simulink model "kaiguangai1108"  (R2016b)
settings: Solver=ode4  StartTime=0.0  StopTime=inf  FixedStep=0.002  RelTol=1e-3  EnableMultiTasking=on
libraries: slrtlib x5
(part 5 of 6)

== stateflow chart kaiguangai1108/Subsystem1/shoudong/Chart3 ==
  state off
    en:
    skhx=0;
    kghx=0;
    gghx=0;
    yjhx=0;
    kgzhiling1=0;
    kgzhiling2=0;
    ggzhiling1=0;
    ggzhiling2=0;
    skyichang=0;
    kgyichang=0;
    sdyichang=0;
    jsyichang=0;
    ggyichang=0;
    yjyichang=0;
  state shoudong
    state songkai [parallel]
      settings: executionOrder=1
      state off
        entry:
        skhx=0;
      state on
        entry:
        skhx=1;
        skt=0;
        skyichang=0;
      state t
        entry:
        skt=skt+0.002;
      state t1
        entry:
        skyichang=1;
      state t2
        entry:
        skt=skt+0.002;
      (default) -> shoudong.songkai.off
      shoudong.songkai.t2 -> shoudong.songkai.off [order 2] : [skdw==1]
      (junction 19) -> shoudong.songkai.off [order 2] : [skdw==1&&skt<=2]
      shoudong.songkai.off -> shoudong.songkai.on : [songkai==1&&yjdw==1]
      shoudong.songkai.on -> (junction 19)
      (junction 19) -> shoudong.songkai.t1 [order 3] : [skt>2]
      shoudong.songkai.t -> (junction 19) : after(1,tick)
      (junction 19) -> shoudong.songkai.t [order 1] : [skdw==0&&skt<=2]
      shoudong.songkai.t1 -> shoudong.songkai.t2
      shoudong.songkai.t2 -> shoudong.songkai.t2 [order 1] : [skdw==0]
    state kaigai [parallel]
      settings: executionOrder=2
      state off
        entry:
        kghx=0;
        kgzhiling1=0;
        kgzhiling2=0；
      state on
        entry:
        kghx=1;
        kgzhiling1=1;
        kgzhiling2=1;
        kgyichang=0;
        kgt=0;
      state t
        entry:
        kgt=kgt+0.002;
      state t1
        entry:
        kgyichang=1;
      state t2
        entry:
        kgt=kgt+0.002;
      (default) -> shoudong.kaigai.off
      shoudong.kaigai.t2 -> shoudong.kaigai.off [order 2] : [kgdw1==1&&kgdw2==1]
      (junction 39) -> shoudong.kaigai.off [order 2] : [kgdw1==1&&kgdw2==1&&kgt<=12]
      shoudong.kaigai.off -> shoudong.kaigai.on : [kaigai==1&&skdw==1]
      shoudong.kaigai.on -> (junction 39)
      (junction 39) -> shoudong.kaigai.t1 [order 3] : [kgt>12]
      shoudong.kaigai.t -> (junction 39) : after(1,tick)
      (junction 39) -> shoudong.kaigai.t [order 1] : [(kgdw1==0||kgdw2==0)&&kgt<=12]
      shoudong.kaigai.t1 -> shoudong.kaigai.t2
      shoudong.kaigai.t2 -> shoudong.kaigai.t2 [order 1] : [kgdw1==0||kgdw2==0]
    state jiesuo_songkai [parallel]
      settings: executionOrder=4
      state off
        entry:
        skhx=0;
      state on
        entry:
        skhx=1;
        jsyichang=0;
        jst=0;
      state t
        entry:
        jst=jst+0.002;
      state t1
        entry:
        jsyichang=1;
      state t2
        entry:
        jst=jst+0.002;
      (default) -> shoudong.jiesuo_songkai.off
      shoudong.jiesuo_songkai.t2 -> shoudong.jiesuo_songkai.off [order 2] : [jsdw==1]
      (junction 60) -> shoudong.jiesuo_songkai.off [order 2] : [skdw==1&&jst<=2]
      shoudong.jiesuo_songkai.off -> shoudong.jiesuo_songkai.on : [jiesuo==1&&sddw==1]
      shoudong.jiesuo_songkai.on -> (junction 60)
      (junction 60) -> shoudong.jiesuo_songkai.t1 [order 3] : [jst>2]
      shoudong.jiesuo_songkai.t -> (junction 60) : after(1,tick)
      (junction 60) -> shoudong.jiesuo_songkai.t [order 1] : [jsdw==0&&jst<=2]
      shoudong.jiesuo_songkai.t1 -> shoudong.jiesuo_songkai.t2
      shoudong.jiesuo_songkai.t2 -> shoudong.jiesuo_songkai.t2 [order 1] : [jsdw==0]
    state suoding_yajin [parallel]
      settings: executionOrder=3
      state off
        entry:
        yjhx=0;
      state on
        entry:
        yjhx=1;
        sdyichang=0;
        sdt=0;
      state t1
        entry:
        sdyichang=1;
      state t2
        entry:
        sdt=sdt+0.002;
      state t
        entry:
        sdt=sdt+0.002;
      (default) -> shoudong.suoding_yajin.off
      shoudong.suoding_yajin.t2 -> shoudong.suoding_yajin.off [order 2] : [sddw==1]
      (junction 48) -> shoudong.suoding_yajin.off [order 2] : [sddw==1&&sdt<=2]
      shoudong.suoding_yajin.off -> shoudong.suoding_yajin.on : [suoding==1&&jsdw==1]
      shoudong.suoding_yajin.on -> (junction 48)
      (junction 48) -> shoudong.suoding_yajin.t1 [order 3] : [sdt>2]
      shoudong.suoding_yajin.t -> (junction 48) : after(1,tick)
      (junction 48) -> shoudong.suoding_yajin.t [order 1] : [sddw==0&&sdt<=2]
      shoudong.suoding_yajin.t1 -> shoudong.suoding_yajin.t2
      shoudong.suoding_yajin.t2 -> shoudong.suoding_yajin.t2 [order 1] : [sddw==0]
    state yajin [parallel]
      settings: executionOrder=6
      state off
        entry:
        yjhx=0;
      state on
        entry:
        yjhx=1;
        yjyichang=0;
        yjt=0;
      state t3
        entry:
        yjyichang=1;
      state t2
        entry:
        yjt=yjt+0.002;
      state t
        entry:
        yjt=yjt+0.002;
      (default) -> shoudong.yajin.off
      shoudong.yajin.t2 -> shoudong.yajin.off [order 2] : [yjdw==1]
      (junction 94) -> shoudong.yajin.off [order 2] : [yjdw==1&&sddw==1&&yjt<=2]
      shoudong.yajin.off -> shoudong.yajin.on : [yajin==1&&skdw==1]
      shoudong.yajin.on -> (junction 94)
      (junction 94) -> t3 [order 3] : [yjt>2]
      shoudong.yajin.t -> (junction 94) : after(1,tick)
      (junction 94) -> shoudong.yajin.t [order 1] : [yjdw==0&&yjt<=2]
      t3 -> shoudong.yajin.t2
      shoudong.yajin.t2 -> shoudong.yajin.t2 [order 1] : [yjdw==0]
    state guangai [parallel]
      settings: executionOrder=5
      state off
        entry:
        gghx=0;
        ggzhiling1=0;
        ggzhiling2=0
      state on
        entry:
        gghx=1;
        ggzhiling1=1;
        ggzhiling2=1;
        ggyichang=0;
        ggt=0;
      state t1
        entry:
        ggyichang=1;
      state t2
        entry:
        ggt=ggt+0.002;
      state t
        entry:
        ggt=ggt+0.002;
      (default) -> shoudong.guangai.off
      shoudong.guangai.t2 -> shoudong.guangai.off [order 2] : [ggdw1==1&&ggdw2==1]
      (junction 81) -> shoudong.guangai.off [order 2] : [ggdw1==1&&ggdw2==1&&ggt<=12]
      shoudong.guangai.off -> shoudong.guangai.on : [guangai==1&&kgdw1==1&&kgdw2==1]
      shoudong.guangai.on -> (junction 81)
      (junction 81) -> shoudong.guangai.t1 [order 3] : [ggt>12]
      shoudong.guangai.t -> (junction 81) : after(1,tick)
      (junction 81) -> shoudong.guangai.t [order 1] : [(ggdw1==0||ggdw2==0)&&ggt<=12]
      shoudong.guangai.t1 -> shoudong.guangai.t2
      shoudong.guangai.t2 -> shoudong.guangai.t2 [order 1] : [ggdw1==0||ggdw2==0]
  state off1
    en:
    skhx=0;
    kghx=0;
    gghx=0;
    yjhx=0;
    skt=0;
    kgt=0;
    sdt=0;
    jst=0;
    ggt=0;
    yjt=0;
    skyichang=0;
    kgyichang=0;
    sdyichang=0;
    jsyichang=0;
    ggyichang=0;
    yjyichang=0;
    kgzhiling1=0;
    kgzhiling2=0;
    ggzhiling1=0;
    ggzhiling2=0;
  (default) -> off
  off -> shoudong : [start==1&&jieshu==0]
  shoudong -> off1 : [jieshu==1]
  data: start input; kgdw1 input; kgdw2 input; ggdw1 input; ggdw2 input; sddw input; jsdw input; yjdw input; skdw input; songkai input; kaigai input; suoding input; jiesuo input; skhx output; kghx output; yjhx output; gghx output; kgzhiling1 output; kgzhiling2 output; ggzhiling1 output; ggzhiling2 output; skt output; kgt output; sdt output; jst output; ggt output; guangai input; yajin input; yjt output; skyichang output; kgyichang output; sdyichang output; jsyichang output; jieshu input; ggyichang output; yjyichang output

== stateflow chart kaiguangai1108/Subsystem1/shoudong/Chart4 ==
  state off
    en:
    skhx=0;
    kghx=0;
    gghx=0;
    yjhx=0;
    kgzhiling1=0;
    kgzhiling2=0;
    ggzhiling1=0;
    ggzhiling2=0;
    skyichang=0;
    kgyichang=0;
    sdyichang=0;
    jsyichang=0;
    ggyichang=0;
    yjyichang=0;
  state shoudong
    state songkai [parallel]
      settings: executionOrder=1
      state off
        entry:
        skhx=0;
      state on
        entry:
        skhx=1;
        skt=0;
        skyichang=0;
      state t
        entry:
        skt=skt+0.002;
      state t1
        entry:
        skyichang=1;
      state t2
        entry:
        skt=skt+0.002;
      (default) -> shoudong.songkai.off
      shoudong.songkai.t2 -> shoudong.songkai.off [order 2] : [skdw==1]
      (junction 19) -> shoudong.songkai.off [order 2] : [skdw==1&&skt<=2]
      shoudong.songkai.off -> shoudong.songkai.on : [songkai==1&&yjdw==1]
      shoudong.songkai.on -> (junction 19)
      (junction 19) -> shoudong.songkai.t1 [order 3] : [skt>2]
      shoudong.songkai.t -> (junction 19) : after(1,tick)
      (junction 19) -> shoudong.songkai.t [order 1] : [skdw==0&&skt<=2]
      shoudong.songkai.t1 -> shoudong.songkai.t2
      shoudong.songkai.t2 -> shoudong.songkai.t2 [order 1] : [skdw==0]
    state kaigai [parallel]
      settings: executionOrder=2
      state off
        entry:
        kghx=0;
        kgzhiling1=0;
        kgzhiling2=0；
      state on
        entry:
        kghx=1;
        kgzhiling1=1;
        kgzhiling2=1;
        kgyichang=0;
        kgt=0;
      state t
        entry:
        kgt=kgt+0.002;
      state t1
        entry:
        kgyichang=1;
      state t2
        entry:
        kgt=kgt+0.002;
      (default) -> shoudong.kaigai.off
      shoudong.kaigai.t2 -> shoudong.kaigai.off [order 2] : [kgdw1==1&&kgdw2==1]
      (junction 39) -> shoudong.kaigai.off [order 2] : [kgdw1==1&&kgdw2==1&&kgt<=12]
      shoudong.kaigai.off -> shoudong.kaigai.on : [kaigai==1&&skdw==1]
      shoudong.kaigai.on -> (junction 39)
      (junction 39) -> shoudong.kaigai.t1 [order 3] : [kgt>12]
      shoudong.kaigai.t -> (junction 39) : after(1,tick)
      (junction 39) -> shoudong.kaigai.t [order 1] : [(kgdw1==0||kgdw2==0)&&kgt<=12]
      shoudong.kaigai.t1 -> shoudong.kaigai.t2
      shoudong.kaigai.t2 -> shoudong.kaigai.t2 [order 1] : [kgdw1==0||kgdw2==0]
    state jiesuo_songkai [parallel]
      settings: executionOrder=4
      state off
        entry:
        skhx=0;
      state on
        entry:
        skhx=1;
        jsyichang=0;
        jst=0;
      state t
        entry:
        jst=jst+0.002;
      state t1
        entry:
        jsyichang=1;
      state t2
        entry:
        jst=jst+0.002;
      (default) -> shoudong.jiesuo_songkai.off
      shoudong.jiesuo_songkai.t2 -> shoudong.jiesuo_songkai.off [order 2] : [jsdw==1]
      (junction 60) -> shoudong.jiesuo_songkai.off [order 2] : [skdw==1&&jst<=2]
      shoudong.jiesuo_songkai.off -> shoudong.jiesuo_songkai.on : [jiesuo==1&&sddw==1]
      shoudong.jiesuo_songkai.on -> (junction 60)
      (junction 60) -> shoudong.jiesuo_songkai.t1 [order 3] : [jst>2]
      shoudong.jiesuo_songkai.t -> (junction 60) : after(1,tick)
      (junction 60) -> shoudong.jiesuo_songkai.t [order 1] : [jsdw==0&&jst<=2]
      shoudong.jiesuo_songkai.t1 -> shoudong.jiesuo_songkai.t2
      shoudong.jiesuo_songkai.t2 -> shoudong.jiesuo_songkai.t2 [order 1] : [jsdw==0]
    state suoding_yajin [parallel]
      settings: executionOrder=3
      state off
        entry:
        yjhx=0;
      state on
        entry:
        yjhx=1;
        sdyichang=0;
        sdt=0;
      state t1
        entry:
        sdyichang=1;
      state t2
        entry:
        sdt=sdt+0.002;
      state t
        entry:
        sdt=sdt+0.002;
      (default) -> shoudong.suoding_yajin.off
      shoudong.suoding_yajin.t2 -> shoudong.suoding_yajin.off [order 2] : [sddw==1]
      (junction 48) -> shoudong.suoding_yajin.off [order 2] : [sddw==1&&sdt<=2]
      shoudong.suoding_yajin.off -> shoudong.suoding_yajin.on : [suoding==1&&jsdw==1]
      shoudong.suoding_yajin.on -> (junction 48)
      (junction 48) -> shoudong.suoding_yajin.t1 [order 3] : [sdt>2]
      shoudong.suoding_yajin.t -> (junction 48) : after(1,tick)
      (junction 48) -> shoudong.suoding_yajin.t [order 1] : [sddw==0&&sdt<=2]
      shoudong.suoding_yajin.t1 -> shoudong.suoding_yajin.t2
      shoudong.suoding_yajin.t2 -> shoudong.suoding_yajin.t2 [order 1] : [sddw==0]
    state yajin [parallel]
      settings: executionOrder=6
      state off
        entry:
        yjhx=0;
      state on
        entry:
        yjhx=1;
        yjyichang=0;
        yjt=0;
      state t3
        entry:
        yjyichang=1;
      state t2
        entry:
        yjt=yjt+0.002;
      state t
        entry:
        yjt=yjt+0.002;
      (default) -> shoudong.yajin.off
      shoudong.yajin.t2 -> shoudong.yajin.off [order 2] : [yjdw==1]
      (junction 94) -> shoudong.yajin.off [order 2] : [yjdw==1&&sddw==1&&yjt<=2]
      shoudong.yajin.off -> shoudong.yajin.on : [yajin==1&&skdw==1]
      shoudong.yajin.on -> (junction 94)
      (junction 94) -> t3 [order 3] : [yjt>2]
      shoudong.yajin.t -> (junction 94) : after(1,tick)
      (junction 94) -> shoudong.yajin.t [order 1] : [yjdw==0&&yjt<=2]
      t3 -> shoudong.yajin.t2
      shoudong.yajin.t2 -> shoudong.yajin.t2 [order 1] : [yjdw==0]
    state guangai [parallel]
      settings: executionOrder=5
      state off
        entry:
        gghx=0;
        ggzhiling1=0;
        ggzhiling2=0
      state on
        entry:
        gghx=1;
        ggzhiling1=1;
        ggzhiling2=1;
        ggyichang=0;
        ggt=0;
      state t1
        entry:
        ggyichang=1;
      state t2
        entry:
        ggt=ggt+0.002;
      state t
        entry:
        ggt=ggt+0.002;
      (default) -> shoudong.guangai.off
      shoudong.guangai.t2 -> shoudong.guangai.off [order 2] : [ggdw1==1&&ggdw2==1]
      (junction 81) -> shoudong.guangai.off [order 2] : [ggdw1==1&&ggdw2==1&&ggt<=12]
      shoudong.guangai.off -> shoudong.guangai.on : [guangai==1&&kgdw1==1&&kgdw2==1]
      shoudong.guangai.on -> (junction 81)
      (junction 81) -> shoudong.guangai.t1 [order 3] : [ggt>12]
      shoudong.guangai.t -> (junction 81) : after(1,tick)
      (junction 81) -> shoudong.guangai.t [order 1] : [(ggdw1==0||ggdw2==0)&&ggt<=12]
      shoudong.guangai.t1 -> shoudong.guangai.t2
      shoudong.guangai.t2 -> shoudong.guangai.t2 [order 1] : [ggdw1==0||ggdw2==0]
  state off1
    en:
    skhx=0;
    kghx=0;
    gghx=0;
    yjhx=0;
    skt=0;
    kgt=0;
    sdt=0;
    jst=0;
    ggt=0;
    yjt=0;
    skyichang=0;
    kgyichang=0;
    sdyichang=0;
    jsyichang=0;
    ggyichang=0;
    yjyichang=0;
    kgzhiling1=0;
    kgzhiling2=0;
    ggzhiling1=0;
    ggzhiling2=0;
  (default) -> off
  off -> shoudong : [start==1&&jieshu==0]
  shoudong -> off1 : [jieshu==1]
  data: start input; kgdw1 input; kgdw2 input; ggdw1 input; ggdw2 input; sddw input; jsdw input; yjdw input; skdw input; songkai input; kaigai input; suoding input; jiesuo input; skhx output; kghx output; yjhx output; gghx output; kgzhiling1 output; kgzhiling2 output; ggzhiling1 output; ggzhiling2 output; skt output; kgt output; sdt output; jst output; ggt output; guangai input; yajin input; yjt output; skyichang output; kgyichang output; sdyichang output; jsyichang output; jieshu input; ggyichang output; yjyichang output

== stateflow chart kaiguangai1108/Subsystem1/shoudong/Chart5 ==
  state off
    en:
    skhx=0;
    kghx=0;
    gghx=0;
    yjhx=0;
    kgzhiling1=0;
    kgzhiling2=0;
    ggzhiling1=0;
    ggzhiling2=0;
    skyichang=0;
    kgyichang=0;
    sdyichang=0;
    jsyichang=0;
    ggyichang=0;
    yjyichang=0;
  state shoudong
    state songkai [parallel]
      settings: executionOrder=1
      state off
        entry:
        skhx=0;
      state on
        entry:
        skhx=1;
        skt=0;
        skyichang=0;
      state t
        entry:
        skt=skt+0.002;
      state t1
        entry:
        skyichang=1;
      state t2
        entry:
        skt=skt+0.002;
      (default) -> shoudong.songkai.off
      shoudong.songkai.t2 -> shoudong.songkai.off [order 2] : [skdw==1]
      (junction 19) -> shoudong.songkai.off [order 2] : [skdw==1&&skt<=2]
      shoudong.songkai.off -> shoudong.songkai.on : [songkai==1&&yjdw==1]
      shoudong.songkai.on -> (junction 19)
      (junction 19) -> shoudong.songkai.t1 [order 3] : [skt>2]
      shoudong.songkai.t -> (junction 19) : after(1,tick)
      (junction 19) -> shoudong.songkai.t [order 1] : [skdw==0&&skt<=2]
      shoudong.songkai.t1 -> shoudong.songkai.t2
      shoudong.songkai.t2 -> shoudong.songkai.t2 [order 1] : [skdw==0]
    state kaigai [parallel]
      settings: executionOrder=2
      state off
        entry:
        kghx=0;
        kgzhiling1=0;
        kgzhiling2=0；
      state on
        entry:
        kghx=1;
        kgzhiling1=1;
        kgzhiling2=1;
        kgyichang=0;
        kgt=0;
      state t
        entry:
        kgt=kgt+0.002;
      state t1
        entry:
        kgyichang=1;
      state t2
        entry:
        kgt=kgt+0.002;
      (default) -> shoudong.kaigai.off
      shoudong.kaigai.t2 -> shoudong.kaigai.off [order 2] : [kgdw1==1&&kgdw2==1]
      (junction 39) -> shoudong.kaigai.off [order 2] : [kgdw1==1&&kgdw2==1&&kgt<=12]
      shoudong.kaigai.off -> shoudong.kaigai.on : [kaigai==1&&skdw==1]
      shoudong.kaigai.on -> (junction 39)
      (junction 39) -> shoudong.kaigai.t1 [order 3] : [kgt>12]
      shoudong.kaigai.t -> (junction 39) : after(1,tick)
      (junction 39) -> shoudong.kaigai.t [order 1] : [(kgdw1==0||kgdw2==0)&&kgt<=12]
      shoudong.kaigai.t1 -> shoudong.kaigai.t2
      shoudong.kaigai.t2 -> shoudong.kaigai.t2 [order 1] : [kgdw1==0||kgdw2==0]
    state jiesuo_songkai [parallel]
      settings: executionOrder=4
      state off
        entry:
        skhx=0;
      state on
        entry:
        skhx=1;
        jsyichang=0;
        jst=0;
      state t
        entry:
        jst=jst+0.002;
      state t1
        entry:
        jsyichang=1;
      state t2
        entry:
        jst=jst+0.002;
      (default) -> shoudong.jiesuo_songkai.off
      shoudong.jiesuo_songkai.t2 -> shoudong.jiesuo_songkai.off [order 2] : [jsdw==1]
      (junction 60) -> shoudong.jiesuo_songkai.off [order 2] : [skdw==1&&jst<=2]
      shoudong.jiesuo_songkai.off -> shoudong.jiesuo_songkai.on : [jiesuo==1&&sddw==1]
      shoudong.jiesuo_songkai.on -> (junction 60)
      (junction 60) -> shoudong.jiesuo_songkai.t1 [order 3] : [jst>2]
      shoudong.jiesuo_songkai.t -> (junction 60) : after(1,tick)
      (junction 60) -> shoudong.jiesuo_songkai.t [order 1] : [jsdw==0&&jst<=2]
      shoudong.jiesuo_songkai.t1 -> shoudong.jiesuo_songkai.t2
      shoudong.jiesuo_songkai.t2 -> shoudong.jiesuo_songkai.t2 [order 1] : [jsdw==0]
    state suoding_yajin [parallel]
      settings: executionOrder=3
      state off
        entry:
        yjhx=0;
      state on
        entry:
        yjhx=1;
        sdyichang=0;
        sdt=0;
      state t1
        entry:
        sdyichang=1;
      state t2
        entry:
        sdt=sdt+0.002;
      state t
        entry:
        sdt=sdt+0.002;
      (default) -> shoudong.suoding_yajin.off
      shoudong.suoding_yajin.t2 -> shoudong.suoding_yajin.off [order 2] : [sddw==1]
      (junction 48) -> shoudong.suoding_yajin.off [order 2] : [sddw==1&&sdt<=2]
      shoudong.suoding_yajin.off -> shoudong.suoding_yajin.on : [suoding==1&&jsdw==1]
      shoudong.suoding_yajin.on -> (junction 48)
      (junction 48) -> shoudong.suoding_yajin.t1 [order 3] : [sdt>2]
      shoudong.suoding_yajin.t -> (junction 48) : after(1,tick)
      (junction 48) -> shoudong.suoding_yajin.t [order 1] : [sddw==0&&sdt<=2]
      shoudong.suoding_yajin.t1 -> shoudong.suoding_yajin.t2
      shoudong.suoding_yajin.t2 -> shoudong.suoding_yajin.t2 [order 1] : [sddw==0]
    state yajin [parallel]
      settings: executionOrder=6
      state off
        entry:
        yjhx=0;
      state on
        entry:
        yjhx=1;
        yjyichang=0;
        yjt=0;
      state t3
        entry:
        yjyichang=1;
      state t2
        entry:
        yjt=yjt+0.002;
      state t
        entry:
        yjt=yjt+0.002;
      (default) -> shoudong.yajin.off
      shoudong.yajin.t2 -> shoudong.yajin.off [order 2] : [yjdw==1]
      (junction 94) -> shoudong.yajin.off [order 2] : [yjdw==1&&sddw==1&&yjt<=2]
      shoudong.yajin.off -> shoudong.yajin.on : [yajin==1&&skdw==1]
      shoudong.yajin.on -> (junction 94)
      (junction 94) -> t3 [order 3] : [yjt>2]
      shoudong.yajin.t -> (junction 94) : after(1,tick)
      (junction 94) -> shoudong.yajin.t [order 1] : [yjdw==0&&yjt<=2]
      t3 -> shoudong.yajin.t2
      shoudong.yajin.t2 -> shoudong.yajin.t2 [order 1] : [yjdw==0]
    state guangai [parallel]
      settings: executionOrder=5
      state off
        entry:
        gghx=0;
        ggzhiling1=0;
        ggzhiling2=0
      state on
        entry:
        gghx=1;
        ggzhiling1=1;
        ggzhiling2=1;
        ggyichang=0;
        ggt=0;
      state t1
        entry:
        ggyichang=1;
      state t2
        entry:
        ggt=ggt+0.002;
      state t
        entry:
        ggt=ggt+0.002;
      (default) -> shoudong.guangai.off
      shoudong.guangai.t2 -> shoudong.guangai.off [order 2] : [ggdw1==1&&ggdw2==1]
      (junction 81) -> shoudong.guangai.off [order 2] : [ggdw1==1&&ggdw2==1&&ggt<=12]
      shoudong.guangai.off -> shoudong.guangai.on : [guangai==1&&kgdw1==1&&kgdw2==1]
      shoudong.guangai.on -> (junction 81)
      (junction 81) -> shoudong.guangai.t1 [order 3] : [ggt>12]
      shoudong.guangai.t -> (junction 81) : after(1,tick)
      (junction 81) -> shoudong.guangai.t [order 1] : [(ggdw1==0||ggdw2==0)&&ggt<=12]
      shoudong.guangai.t1 -> shoudong.guangai.t2
      shoudong.guangai.t2 -> shoudong.guangai.t2 [order 1] : [ggdw1==0||ggdw2==0]
  state off1
    en:
    skhx=0;
    kghx=0;
    gghx=0;
    yjhx=0;
    skt=0;
    kgt=0;
    sdt=0;
    jst=0;
    ggt=0;
    yjt=0;
    skyichang=0;
    kgyichang=0;
    sdyichang=0;
    jsyichang=0;
    ggyichang=0;
    yjyichang=0;
    kgzhiling1=0;
    kgzhiling2=0;
    ggzhiling1=0;
    ggzhiling2=0;
  (default) -> off
  off -> shoudong : [start==1&&jieshu==0]
  shoudong -> off1 : [jieshu==1]
  data: start input; kgdw1 input; kgdw2 input; ggdw1 input; ggdw2 input; sddw input; jsdw input; yjdw input; skdw input; songkai input; kaigai input; suoding input; jiesuo input; skhx output; kghx output; yjhx output; gghx output; kgzhiling1 output; kgzhiling2 output; ggzhiling1 output; ggzhiling2 output; skt output; kgt output; sdt output; jst output; ggt output; guangai input; yajin input; yjt output; skyichang output; kgyichang output; sdyichang output; jsyichang output; jieshu input; ggyichang output; yjyichang output

== stateflow chart kaiguangai1108/Subsystem1/shoudong/Chart6 ==
  state off
    en:
    skhx=0;
    kghx=0;
    gghx=0;
    yjhx=0;
    kgzhiling1=0;
    kgzhiling2=0;
    ggzhiling1=0;
    ggzhiling2=0;
    skyichang=0;
    kgyichang=0;
    sdyichang=0;
    jsyichang=0;
    ggyichang=0;
    yjyichang=0;
  state shoudong
    state songkai [parallel]
      settings: executionOrder=1
      state off
        entry:
        skhx=0;
      state on
        entry:
        skhx=1;
        skt=0;
        skyichang=0;
      state t
        entry:
        skt=skt+0.002;
      state t1
        entry:
        skyichang=1;
      state t2
        entry:
        skt=skt+0.002;
      (default) -> shoudong.songkai.off
      shoudong.songkai.t2 -> shoudong.songkai.off [order 2] : [skdw==1]
      (junction 19) -> shoudong.songkai.off [order 2] : [skdw==1&&skt<=2]
      shoudong.songkai.off -> shoudong.songkai.on : [songkai==1&&yjdw==1]
      shoudong.songkai.on -> (junction 19)
      (junction 19) -> shoudong.songkai.t1 [order 3] : [skt>2]
      shoudong.songkai.t -> (junction 19) : after(1,tick)
      (junction 19) -> shoudong.songkai.t [order 1] : [skdw==0&&skt<=2]
      shoudong.songkai.t1 -> shoudong.songkai.t2
      shoudong.songkai.t2 -> shoudong.songkai.t2 [order 1] : [skdw==0]
    state kaigai [parallel]
      settings: executionOrder=2
      state off
        entry:
        kghx=0;
        kgzhiling1=0;
        kgzhiling2=0；
      state on
        entry:
        kghx=1;
        kgzhiling1=1;
        kgzhiling2=1;
        kgyichang=0;
        kgt=0;
      state t
        entry:
        kgt=kgt+0.002;
      state t1
        entry:
        kgyichang=1;
      state t2
        entry:
        kgt=kgt+0.002;
      (default) -> shoudong.kaigai.off
      shoudong.kaigai.t2 -> shoudong.kaigai.off [order 2] : [kgdw1==1&&kgdw2==1]
      (junction 39) -> shoudong.kaigai.off [order 2] : [kgdw1==1&&kgdw2==1&&kgt<=12]
      shoudong.kaigai.off -> shoudong.kaigai.on : [kaigai==1&&skdw==1]
      shoudong.kaigai.on -> (junction 39)
      (junction 39) -> shoudong.kaigai.t1 [order 3] : [kgt>12]
      shoudong.kaigai.t -> (junction 39) : after(1,tick)
      (junction 39) -> shoudong.kaigai.t [order 1] : [(kgdw1==0||kgdw2==0)&&kgt<=12]
      shoudong.kaigai.t1 -> shoudong.kaigai.t2
      shoudong.kaigai.t2 -> shoudong.kaigai.t2 [order 1] : [kgdw1==0||kgdw2==0]
    state jiesuo_songkai [parallel]
      settings: executionOrder=4
      state off
        entry:
        skhx=0;
      state on
        entry:
        skhx=1;
        jsyichang=0;
        jst=0;
      state t
        entry:
        jst=jst+0.002;
      state t1
        entry:
        jsyichang=1;
      state t2
        entry:
        jst=jst+0.002;
      (default) -> shoudong.jiesuo_songkai.off
      shoudong.jiesuo_songkai.t2 -> shoudong.jiesuo_songkai.off [order 2] : [jsdw==1]
      (junction 60) -> shoudong.jiesuo_songkai.off [order 2] : [skdw==1&&jst<=2]
      shoudong.jiesuo_songkai.off -> shoudong.jiesuo_songkai.on : [jiesuo==1&&sddw==1]
      shoudong.jiesuo_songkai.on -> (junction 60)
      (junction 60) -> shoudong.jiesuo_songkai.t1 [order 3] : [jst>2]
      shoudong.jiesuo_songkai.t -> (junction 60) : after(1,tick)
      (junction 60) -> shoudong.jiesuo_songkai.t [order 1] : [jsdw==0&&jst<=2]
      shoudong.jiesuo_songkai.t1 -> shoudong.jiesuo_songkai.t2
      shoudong.jiesuo_songkai.t2 -> shoudong.jiesuo_songkai.t2 [order 1] : [jsdw==0]
    state suoding_yajin [parallel]
      settings: executionOrder=3
      state off
        entry:
        yjhx=0;
      state on
        entry:
        yjhx=1;
        sdyichang=0;
        sdt=0;
      state t1
        entry:
        sdyichang=1;
      state t2
        entry:
        sdt=sdt+0.002;
      state t
        entry:
        sdt=sdt+0.002;
      (default) -> shoudong.suoding_yajin.off
      shoudong.suoding_yajin.t2 -> shoudong.suoding_yajin.off [order 2] : [sddw==1]
      (junction 48) -> shoudong.suoding_yajin.off [order 2] : [sddw==1&&sdt<=2]
      shoudong.suoding_yajin.off -> shoudong.suoding_yajin.on : [suoding==1&&jsdw==1]
      shoudong.suoding_yajin.on -> (junction 48)
      (junction 48) -> shoudong.suoding_yajin.t1 [order 3] : [sdt>2]
      shoudong.suoding_yajin.t -> (junction 48) : after(1,tick)
      (junction 48) -> shoudong.suoding_yajin.t [order 1] : [sddw==0&&sdt<=2]
      shoudong.suoding_yajin.t1 -> shoudong.suoding_yajin.t2
      shoudong.suoding_yajin.t2 -> shoudong.suoding_yajin.t2 [order 1] : [sddw==0]
    state yajin [parallel]
      settings: executionOrder=6
      state off
        entry:
        yjhx=0;
      state on
        entry:
        yjhx=1;
        yjyichang=0;
        yjt=0;
      state t3
        entry:
        yjyichang=1;
      state t2
        entry:
        yjt=yjt+0.002;
      state t
        entry:
        yjt=yjt+0.002;
      (default) -> shoudong.yajin.off
      shoudong.yajin.t2 -> shoudong.yajin.off [order 2] : [yjdw==1]
      (junction 94) -> shoudong.yajin.off [order 2] : [yjdw==1&&sddw==1&&yjt<=2]
      shoudong.yajin.off -> shoudong.yajin.on : [yajin==1&&skdw==1]
      shoudong.yajin.on -> (junction 94)
      (junction 94) -> t3 [order 3] : [yjt>2]
      shoudong.yajin.t -> (junction 94) : after(1,tick)
      (junction 94) -> shoudong.yajin.t [order 1] : [yjdw==0&&yjt<=2]
      t3 -> shoudong.yajin.t2
      shoudong.yajin.t2 -> shoudong.yajin.t2 [order 1] : [yjdw==0]
    state guangai [parallel]
      settings: executionOrder=5
      state off
        entry:
        gghx=0;
        ggzhiling1=0;
        ggzhiling2=0
      state on
        entry:
        gghx=1;
        ggzhiling1=1;
        ggzhiling2=1;
        ggyichang=0;
        ggt=0;
      state t1
        entry:
        ggyichang=1;
      state t2
        entry:
        ggt=ggt+0.002;
      state t
        entry:
        ggt=ggt+0.002;
      (default) -> shoudong.guangai.off
      shoudong.guangai.t2 -> shoudong.guangai.off [order 2] : [ggdw1==1&&ggdw2==1]
      (junction 81) -> shoudong.guangai.off [order 2] : [ggdw1==1&&ggdw2==1&&ggt<=12]
      shoudong.guangai.off -> shoudong.guangai.on : [guangai==1&&kgdw1==1&&kgdw2==1]
      shoudong.guangai.on -> (junction 81)
      (junction 81) -> shoudong.guangai.t1 [order 3] : [ggt>12]
      shoudong.guangai.t -> (junction 81) : after(1,tick)
      (junction 81) -> shoudong.guangai.t [order 1] : [(ggdw1==0||ggdw2==0)&&ggt<=12]
      shoudong.guangai.t1 -> shoudong.guangai.t2
      shoudong.guangai.t2 -> shoudong.guangai.t2 [order 1] : [ggdw1==0||ggdw2==0]
  state off1
    en:
    skhx=0;
    kghx=0;
    gghx=0;
    yjhx=0;
    skt=0;
    kgt=0;
    sdt=0;
    jst=0;
    ggt=0;
    yjt=0;
    skyichang=0;
    kgyichang=0;
    sdyichang=0;
    jsyichang=0;
    ggyichang=0;
    yjyichang=0;
    kgzhiling1=0;
    kgzhiling2=0;
    ggzhiling1=0;
    ggzhiling2=0;
  (default) -> off
  off -> shoudong : [start==1&&jieshu==0]
  shoudong -> off1 : [jieshu==1]
  data: start input; kgdw1 input; kgdw2 input; ggdw1 input; ggdw2 input; sddw input; jsdw input; yjdw input; skdw input; songkai input; kaigai input; suoding input; jiesuo input; skhx output; kghx output; yjhx output; gghx output; kgzhiling1 output; kgzhiling2 output; ggzhiling1 output; ggzhiling2 output; skt output; kgt output; sdt output; jst output; ggt output; guangai input; yajin input; yjt output; skyichang output; kgyichang output; sdyichang output; jsyichang output; jieshu input; ggyichang output; yjyichang output

== stateflow chart kaiguangai1108/Subsystem1/shoudong/Chart7 ==
  state off
    en:
    skhx=0;
    kghx=0;
    gghx=0;
    yjhx=0;
    kgzhiling1=0;
    kgzhiling2=0;
    ggzhiling1=0;
    ggzhiling2=0;
    skyichang=0;
    kgyichang=0;
    sdyichang=0;
    jsyichang=0;
    ggyichang=0;
    yjyichang=0;
  state shoudong
    state songkai [parallel]
      settings: executionOrder=1
      state off
        entry:
        skhx=0;
      state on
        entry:
        skhx=1;
        skt=0;
        skyichang=0;
      state t
        entry:
        skt=skt+0.002;
      state t1
        entry:
        skyichang=1;
      state t2
        entry:
        skt=skt+0.002;
      (default) -> shoudong.songkai.off
      shoudong.songkai.t2 -> shoudong.songkai.off [order 2] : [skdw==1]
      (junction 19) -> shoudong.songkai.off [order 2] : [skdw==1&&skt<=2]
      shoudong.songkai.off -> shoudong.songkai.on : [songkai==1&&yjdw==1]
      shoudong.songkai.on -> (junction 19)
      (junction 19) -> shoudong.songkai.t1 [order 3] : [skt>2]
      shoudong.songkai.t -> (junction 19) : after(1,tick)
      (junction 19) -> shoudong.songkai.t [order 1] : [skdw==0&&skt<=2]
      shoudong.songkai.t1 -> shoudong.songkai.t2
      shoudong.songkai.t2 -> shoudong.songkai.t2 [order 1] : [skdw==0]
    state kaigai [parallel]
      settings: executionOrder=2
      state off
        entry:
        kghx=0;
        kgzhiling1=0;
        kgzhiling2=0；
      state on
        entry:
        kghx=1;
        kgzhiling1=1;
        kgzhiling2=1;
        kgyichang=0;
        kgt=0;
      state t
        entry:
        kgt=kgt+0.002;
      state t1
        entry:
        kgyichang=1;
      state t2
        entry:
        kgt=kgt+0.002;
      (default) -> shoudong.kaigai.off
      shoudong.kaigai.t2 -> shoudong.kaigai.off [order 2] : [kgdw1==1&&kgdw2==1]
      (junction 39) -> shoudong.kaigai.off [order 2] : [kgdw1==1&&kgdw2==1&&kgt<=12]
      shoudong.kaigai.off -> shoudong.kaigai.on : [kaigai==1&&skdw==1]
      shoudong.kaigai.on -> (junction 39)
      (junction 39) -> shoudong.kaigai.t1 [order 3] : [kgt>12]
      shoudong.kaigai.t -> (junction 39) : after(1,tick)
      (junction 39) -> shoudong.kaigai.t [order 1] : [(kgdw1==0||kgdw2==0)&&kgt<=12]
      shoudong.kaigai.t1 -> shoudong.kaigai.t2
      shoudong.kaigai.t2 -> shoudong.kaigai.t2 [order 1] : [kgdw1==0||kgdw2==0]
    state jiesuo_songkai [parallel]
      settings: executionOrder=4
      state off
        entry:
        skhx=0;
      state on
        entry:
        skhx=1;
        jsyichang=0;
        jst=0;
      state t
        entry:
        jst=jst+0.002;
      state t1
        entry:
        jsyichang=1;
      state t2
        entry:
        jst=jst+0.002;
      (default) -> shoudong.jiesuo_songkai.off
      shoudong.jiesuo_songkai.t2 -> shoudong.jiesuo_songkai.off [order 2] : [jsdw==1]
      (junction 60) -> shoudong.jiesuo_songkai.off [order 2] : [skdw==1&&jst<=2]
      shoudong.jiesuo_songkai.off -> shoudong.jiesuo_songkai.on : [jiesuo==1&&sddw==1]
      shoudong.jiesuo_songkai.on -> (junction 60)
      (junction 60) -> shoudong.jiesuo_songkai.t1 [order 3] : [jst>2]
      shoudong.jiesuo_songkai.t -> (junction 60) : after(1,tick)
      (junction 60) -> shoudong.jiesuo_songkai.t [order 1] : [jsdw==0&&jst<=2]
      shoudong.jiesuo_songkai.t1 -> shoudong.jiesuo_songkai.t2
      shoudong.jiesuo_songkai.t2 -> shoudong.jiesuo_songkai.t2 [order 1] : [jsdw==0]
    state suoding_yajin [parallel]
      settings: executionOrder=3
      state off
        entry:
        yjhx=0;
      state on
        entry:
        yjhx=1;
        sdyichang=0;
        sdt=0;
      state t1
        entry:
        sdyichang=1;
      state t2
        entry:
        sdt=sdt+0.002;
      state t
        entry:
        sdt=sdt+0.002;
      (default) -> shoudong.suoding_yajin.off
      shoudong.suoding_yajin.t2 -> shoudong.suoding_yajin.off [order 2] : [sddw==1]
      (junction 48) -> shoudong.suoding_yajin.off [order 2] : [sddw==1&&sdt<=2]
      shoudong.suoding_yajin.off -> shoudong.suoding_yajin.on : [suoding==1&&jsdw==1]
      shoudong.suoding_yajin.on -> (junction 48)
      (junction 48) -> shoudong.suoding_yajin.t1 [order 3] : [sdt>2]
      shoudong.suoding_yajin.t -> (junction 48) : after(1,tick)
      (junction 48) -> shoudong.suoding_yajin.t [order 1] : [sddw==0&&sdt<=2]
      shoudong.suoding_yajin.t1 -> shoudong.suoding_yajin.t2
      shoudong.suoding_yajin.t2 -> shoudong.suoding_yajin.t2 [order 1] : [sddw==0]
    state yajin [parallel]
      settings: executionOrder=6
      state off
        entry:
        yjhx=0;
      state on
        entry:
        yjhx=1;
        yjyichang=0;
        yjt=0;
      state t3
        entry:
        yjyichang=1;
      state t2
        entry:
        yjt=yjt+0.002;
      state t
        entry:
        yjt=yjt+0.002;
      (default) -> shoudong.yajin.off
      shoudong.yajin.t2 -> shoudong.yajin.off [order 2] : [yjdw==1]
      (junction 94) -> shoudong.yajin.off [order 2] : [yjdw==1&&sddw==1&&yjt<=2]
      shoudong.yajin.off -> shoudong.yajin.on : [yajin==1&&skdw==1]
      shoudong.yajin.on -> (junction 94)
      (junction 94) -> t3 [order 3] : [yjt>2]
      shoudong.yajin.t -> (junction 94) : after(1,tick)
      (junction 94) -> shoudong.yajin.t [order 1] : [yjdw==0&&yjt<=2]
      t3 -> shoudong.yajin.t2
      shoudong.yajin.t2 -> shoudong.yajin.t2 [order 1] : [yjdw==0]
    state guangai [parallel]
      settings: executionOrder=5
      state off
        entry:
        gghx=0;
        ggzhiling1=0;
        ggzhiling2=0
      state on
        entry:
        gghx=1;
        ggzhiling1=1;
        ggzhiling2=1;
        ggyichang=0;
        ggt=0;
      state t1
        entry:
        ggyichang=1;
      state t2
        entry:
        ggt=ggt+0.002;
      state t
        entry:
        ggt=ggt+0.002;
      (default) -> shoudong.guangai.off
      shoudong.guangai.t2 -> shoudong.guangai.off [order 2] : [ggdw1==1&&ggdw2==1]
      (junction 81) -> shoudong.guangai.off [order 2] : [ggdw1==1&&ggdw2==1&&ggt<=12]
      shoudong.guangai.off -> shoudong.guangai.on : [guangai==1&&kgdw1==1&&kgdw2==1]
      shoudong.guangai.on -> (junction 81)
      (junction 81) -> shoudong.guangai.t1 [order 3] : [ggt>12]
      shoudong.guangai.t -> (junction 81) : after(1,tick)
      (junction 81) -> shoudong.guangai.t [order 1] : [(ggdw1==0||ggdw2==0)&&ggt<=12]
      shoudong.guangai.t1 -> shoudong.guangai.t2
      shoudong.guangai.t2 -> shoudong.guangai.t2 [order 1] : [ggdw1==0||ggdw2==0]
  state off1
    en:
    skhx=0;
    kghx=0;
    gghx=0;
    yjhx=0;
    skt=0;
    kgt=0;
    sdt=0;
    jst=0;
    ggt=0;
    yjt=0;
    skyichang=0;
    kgyichang=0;
    sdyichang=0;
    jsyichang=0;
    ggyichang=0;
    yjyichang=0;
    kgzhiling1=0;
    kgzhiling2=0;
    ggzhiling1=0;
    ggzhiling2=0;
  (default) -> off
  off -> shoudong : [start==1&&jieshu==0]
  shoudong -> off1 : [jieshu==1]
  data: start input; kgdw1 input; kgdw2 input; ggdw1 input; ggdw2 input; sddw input; jsdw input; yjdw input; skdw input; songkai input; kaigai input; suoding input; jiesuo input; skhx output; kghx output; yjhx output; gghx output; kgzhiling1 output; kgzhiling2 output; ggzhiling1 output; ggzhiling2 output; skt output; kgt output; sdt output; jst output; ggt output; guangai input; yajin input; yjt output; skyichang output; kgyichang output; sdyichang output; jsyichang output; jieshu input; ggyichang output; yjyichang output

== stateflow chart kaiguangai1108/tiaoshimoshi/jinjichuli1 ==
  state MANUAL
    state kaigai [parallel]
      settings: executionOrder=1
      state A
        entry:kghx=0;
      state on
        entry:kghx=1;
      (default) -> MANUAL.kaigai.A
      MANUAL.kaigai.on -> MANUAL.kaigai.A : [kaigai==0]
      MANUAL.kaigai.A -> MANUAL.kaigai.on : [kaigai==1]
    state guangai [parallel]
      settings: executionOrder=2
      state A
        entry:gghx=0;
      state on
        entry:gghx=1;
      (default) -> MANUAL.guangai.A
      MANUAL.guangai.on -> MANUAL.guangai.A : [guangai==0]
      MANUAL.guangai.A -> MANUAL.guangai.on : [guangai==1]
    state songkai [parallel]
      settings: executionOrder=3
      state A
        entry:skhx=0;
      state on
        entry:skhx=1;
      (default) -> MANUAL.songkai.A
      MANUAL.songkai.on -> MANUAL.songkai.A : [songkai==0]
      MANUAL.songkai.A -> MANUAL.songkai.on : [songkai==1]
    state yajin [parallel]
      settings: executionOrder=4
      state A
        entry:yjhx=0;
      state on
        entry:yjhx=1;
      (default) -> MANUAL.yajin.A
      MANUAL.yajin.on -> MANUAL.yajin.A : [yajin==0]
      MANUAL.yajin.A -> MANUAL.yajin.on : [yajin==1]
    state suoding [parallel]
      settings: executionOrder=5
      state A
        entry:yjhx=0;
      state on
        entry:yjhx=1;
      (default) -> MANUAL.suoding.A
      MANUAL.suoding.on -> MANUAL.suoding.A : [suoding==0]
      MANUAL.suoding.A -> MANUAL.suoding.on : [suoding==1]
    state jiesuo [parallel]
      settings: executionOrder=6
      state A
        entry:skhx=0;
      state on
        entry:skhx=1;
      (default) -> MANUAL.jiesuo.A
      MANUAL.jiesuo.on -> MANUAL.jiesuo.A : [jiesuo==0]
      MANUAL.jiesuo.A -> MANUAL.jiesuo.on : [jiesuo==1]
  state off1
  state on1
    entry:
    skhx=0;
    kghx=0;
    yjhx=0;
    gghx=0;
  state end
    en:
    skhx=0;
    kghx=0;
    yjhx=0;
    gghx=0
  (default) -> off1
  off1 -> on1 : [tiaoshi==1]
  on1 -> MANUAL : after(500,tick)
  MANUAL -> end : [jiting==1]
  data: skhx output double; kghx output double; tiaoshi input double; songkai input; kaigai input; suoding input; jiesuo input; guangai input; yajin input; jiting input; yjhx output double; gghx output double

== stateflow chart kaiguangai1108/tiaoshimoshi/jinjichuli ==
  state MANUAL
    state kaigai [parallel]
      settings: executionOrder=1
      state A
        entry:kghx=0;
      state on
        entry:kghx=1;
      (default) -> MANUAL.kaigai.A
      MANUAL.kaigai.on -> MANUAL.kaigai.A : [kaigai==0]
      MANUAL.kaigai.A -> MANUAL.kaigai.on : [kaigai==1]
    state guangai [parallel]
      settings: executionOrder=2
      state A
        entry:gghx=0;
      state on
        entry:gghx=1;
      (default) -> MANUAL.guangai.A
      MANUAL.guangai.on -> MANUAL.guangai.A : [guangai==0]
      MANUAL.guangai.A -> MANUAL.guangai.on : [guangai==1]
    state songkai [parallel]
      settings: executionOrder=3
      state A
        entry:skhx=0;
      state on
        entry:skhx=1;
      (default) -> MANUAL.songkai.A
      MANUAL.songkai.on -> MANUAL.songkai.A : [songkai==0]
      MANUAL.songkai.A -> MANUAL.songkai.on : [songkai==1]
    state yajin [parallel]
      settings: executionOrder=4
      state A
        entry:yjhx=0;
      state on
        entry:yjhx=1;
      (default) -> MANUAL.yajin.A
      MANUAL.yajin.on -> MANUAL.yajin.A : [yajin==0]
      MANUAL.yajin.A -> MANUAL.yajin.on : [yajin==1]
    state suoding [parallel]
      settings: executionOrder=5
      state A
        entry:yjhx=0;
      state on
        entry:yjhx=1;
      (default) -> MANUAL.suoding.A
      MANUAL.suoding.on -> MANUAL.suoding.A : [suoding==0]
      MANUAL.suoding.A -> MANUAL.suoding.on : [suoding==1]
    state jiesuo [parallel]
      settings: executionOrder=6
      state A
        entry:skhx=0;
      state on
        entry:skhx=1;
      (default) -> MANUAL.jiesuo.A
      MANUAL.jiesuo.on -> MANUAL.jiesuo.A : [jiesuo==0]
      MANUAL.jiesuo.A -> MANUAL.jiesuo.on : [jiesuo==1]
  state off1
  state on1
    entry:
    skhx=0;
    kghx=0;
    yjhx=0;
    gghx=0;
  state end
    en:
    skhx=0;
    kghx=0;
    yjhx=0;
    gghx=0
  (default) -> off1
  off1 -> on1 : [tiaoshi==1]
  on1 -> MANUAL : after(500,tick)
  MANUAL -> end : [jiting==1]
  data: skhx output double; kghx output double; tiaoshi input double; songkai input; kaigai input; suoding input; jiesuo input; guangai input; yajin input; jiting input; yjhx output double; gghx output double

== stateflow chart kaiguangai1108/tiaoshimoshi/jinjichuli2 ==
  state MANUAL
    state kaigai [parallel]
      settings: executionOrder=1
      state A
        entry:kghx=0;
      state on
        entry:kghx=1;
      (default) -> MANUAL.kaigai.A
      MANUAL.kaigai.on -> MANUAL.kaigai.A : [kaigai==0]
      MANUAL.kaigai.A -> MANUAL.kaigai.on : [kaigai==1]
    state guangai [parallel]
      settings: executionOrder=2
      state A
        entry:gghx=0;
      state on
        entry:gghx=1;
      (default) -> MANUAL.guangai.A
      MANUAL.guangai.on -> MANUAL.guangai.A : [guangai==0]
      MANUAL.guangai.A -> MANUAL.guangai.on : [guangai==1]
    state songkai [parallel]
      settings: executionOrder=3
      state A
        entry:skhx=0;
      state on
        entry:skhx=1;
      (default) -> MANUAL.songkai.A
      MANUAL.songkai.on -> MANUAL.songkai.A : [songkai==0]
      MANUAL.songkai.A -> MANUAL.songkai.on : [songkai==1]
    state yajin [parallel]
      settings: executionOrder=4
      state A
        entry:yjhx=0;
      state on
        entry:yjhx=1;
      (default) -> MANUAL.yajin.A
      MANUAL.yajin.on -> MANUAL.yajin.A : [yajin==0]
      MANUAL.yajin.A -> MANUAL.yajin.on : [yajin==1]
    state suoding [parallel]
      settings: executionOrder=5
      state A
        entry:yjhx=0;
      state on
        entry:yjhx=1;
      (default) -> MANUAL.suoding.A
      MANUAL.suoding.on -> MANUAL.suoding.A : [suoding==0]
      MANUAL.suoding.A -> MANUAL.suoding.on : [suoding==1]
    state jiesuo [parallel]
      settings: executionOrder=6
      state A
        entry:skhx=0;
      state on
        entry:skhx=1;
      (default) -> MANUAL.jiesuo.A
      MANUAL.jiesuo.on -> MANUAL.jiesuo.A : [jiesuo==0]
      MANUAL.jiesuo.A -> MANUAL.jiesuo.on : [jiesuo==1]
  state off1
  state on1
    entry:
    skhx=0;
    kghx=0;
    yjhx=0;
    gghx=0;
  state end
    en:
    skhx=0;
    kghx=0;
    yjhx=0;
    gghx=0
  (default) -> off1
  off1 -> on1 : [tiaoshi==1]
  on1 -> MANUAL : after(500,tick)
  MANUAL -> end : [jiting==1]
  data: skhx output double; kghx output double; tiaoshi input double; songkai input; kaigai input; suoding input; jiesuo input; guangai input; yajin input; jiting input; yjhx output double; gghx output double

== stateflow chart kaiguangai1108/tiaoshimoshi/jinjichuli3 ==
  state MANUAL
    state kaigai [parallel]
      settings: executionOrder=1
      state A
        entry:kghx=0;
      state on
        entry:kghx=1;
      (default) -> MANUAL.kaigai.A
      MANUAL.kaigai.on -> MANUAL.kaigai.A : [kaigai==0]
      MANUAL.kaigai.A -> MANUAL.kaigai.on : [kaigai==1]
    state guangai [parallel]
      settings: executionOrder=2
      state A
        entry:gghx=0;
      state on
        entry:gghx=1;
      (default) -> MANUAL.guangai.A
      MANUAL.guangai.on -> MANUAL.guangai.A : [guangai==0]
      MANUAL.guangai.A -> MANUAL.guangai.on : [guangai==1]
    state songkai [parallel]
      settings: executionOrder=3
      state A
        entry:skhx=0;
      state on
        entry:skhx=1;
      (default) -> MANUAL.songkai.A
      MANUAL.songkai.on -> MANUAL.songkai.A : [songkai==0]
      MANUAL.songkai.A -> MANUAL.songkai.on : [songkai==1]
    state yajin [parallel]
      settings: executionOrder=4
      state A
        entry:yjhx=0;
      state on
        entry:yjhx=1;
      (default) -> MANUAL.yajin.A
      MANUAL.yajin.on -> MANUAL.yajin.A : [yajin==0]
      MANUAL.yajin.A -> MANUAL.yajin.on : [yajin==1]
    state suoding [parallel]
      settings: executionOrder=5
      state A
        entry:yjhx=0;
      state on
        entry:yjhx=1;
      (default) -> MANUAL.suoding.A
      MANUAL.suoding.on -> MANUAL.suoding.A : [suoding==0]
      MANUAL.suoding.A -> MANUAL.suoding.on : [suoding==1]
    state jiesuo [parallel]
      settings: executionOrder=6
      state A
        entry:skhx=0;
      state on
        entry:skhx=1;
      (default) -> MANUAL.jiesuo.A
      MANUAL.jiesuo.on -> MANUAL.jiesuo.A : [jiesuo==0]
      MANUAL.jiesuo.A -> MANUAL.jiesuo.on : [jiesuo==1]
  state off1
  state on1
    entry:
    skhx=0;
    kghx=0;
    yjhx=0;
    gghx=0;
  state end
    en:
    skhx=0;
    kghx=0;
    yjhx=0;
    gghx=0
  (default) -> off1
  off1 -> on1 : [tiaoshi==1]
  on1 -> MANUAL : after(500,tick)
  MANUAL -> end : [jiting==1]
  data: skhx output double; kghx output double; tiaoshi input double; songkai input; kaigai input; suoding input; jiesuo input; guangai input; yajin input; jiting input; yjhx output double; gghx output double

== stateflow chart kaiguangai1108/tiaoshimoshi/jinjichuli4 ==
  state MANUAL
    state kaigai [parallel]
      settings: executionOrder=1
      state A
        entry:kghx=0;
      state on
        entry:kghx=1;
      (default) -> MANUAL.kaigai.A
      MANUAL.kaigai.on -> MANUAL.kaigai.A : [kaigai==0]
      MANUAL.kaigai.A -> MANUAL.kaigai.on : [kaigai==1]
    state guangai [parallel]
      settings: executionOrder=2
      state A
        entry:gghx=0;
      state on
        entry:gghx=1;
      (default) -> MANUAL.guangai.A
      MANUAL.guangai.on -> MANUAL.guangai.A : [guangai==0]
      MANUAL.guangai.A -> MANUAL.guangai.on : [guangai==1]
    state songkai [parallel]
      settings: executionOrder=3
      state A
        entry:skhx=0;
      state on
        entry:skhx=1;
      (default) -> MANUAL.songkai.A
      MANUAL.songkai.on -> MANUAL.songkai.A : [songkai==0]
      MANUAL.songkai.A -> MANUAL.songkai.on : [songkai==1]
    state yajin [parallel]
      settings: executionOrder=4
      state A
        entry:yjhx=0;
      state on
        entry:yjhx=1;
      (default) -> MANUAL.yajin.A
      MANUAL.yajin.on -> MANUAL.yajin.A : [yajin==0]
      MANUAL.yajin.A -> MANUAL.yajin.on : [yajin==1]
    state suoding [parallel]
      settings: executionOrder=5
      state A
        entry:yjhx=0;
      state on
        entry:yjhx=1;
      (default) -> MANUAL.suoding.A
      MANUAL.suoding.on -> MANUAL.suoding.A : [suoding==0]
      MANUAL.suoding.A -> MANUAL.suoding.on : [suoding==1]
    state jiesuo [parallel]
      settings: executionOrder=6
      state A
        entry:skhx=0;
      state on
        entry:skhx=1;
      (default) -> MANUAL.jiesuo.A
      MANUAL.jiesuo.on -> MANUAL.jiesuo.A : [jiesuo==0]
      MANUAL.jiesuo.A -> MANUAL.jiesuo.on : [jiesuo==1]
  state off1
  state on1
    entry:
    skhx=0;
    kghx=0;
    yjhx=0;
    gghx=0;
  state end
    en:
    skhx=0;
    kghx=0;
    yjhx=0;
    gghx=0
  (default) -> off1
  off1 -> on1 : [tiaoshi==1]
  on1 -> MANUAL : after(500,tick)
  MANUAL -> end : [jiting==1]
  data: skhx output double; kghx output double; tiaoshi input double; songkai input; kaigai input; suoding input; jiesuo input; guangai input; yajin input; jiting input; yjhx output double; gghx output double

== stateflow chart kaiguangai1108/tiaoshimoshi/jinjichuli5 ==
  state MANUAL
    state kaigai [parallel]
      settings: executionOrder=1
      state A
        entry:kghx=0;
      state on
        entry:kghx=1;
      (default) -> MANUAL.kaigai.A
      MANUAL.kaigai.on -> MANUAL.kaigai.A : [kaigai==0]
      MANUAL.kaigai.A -> MANUAL.kaigai.on : [kaigai==1]
    state guangai [parallel]
      settings: executionOrder=2
      state A
        entry:gghx=0;
      state on
        entry:gghx=1;
      (default) -> MANUAL.guangai.A
      MANUAL.guangai.on -> MANUAL.guangai.A : [guangai==0]
      MANUAL.guangai.A -> MANUAL.guangai.on : [guangai==1]
    state songkai [parallel]
      settings: executionOrder=3
      state A
        entry:skhx=0;
      state on
        entry:skhx=1;
      (default) -> MANUAL.songkai.A
      MANUAL.songkai.on -> MANUAL.songkai.A : [songkai==0]
      MANUAL.songkai.A -> MANUAL.songkai.on : [songkai==1]
    state yajin [parallel]
      settings: executionOrder=4
      state A
        entry:yjhx=0;
      state on
        entry:yjhx=1;
      (default) -> MANUAL.yajin.A
      MANUAL.yajin.on -> MANUAL.yajin.A : [yajin==0]
      MANUAL.yajin.A -> MANUAL.yajin.on : [yajin==1]
    state suoding [parallel]
      settings: executionOrder=5
      state A
        entry:yjhx=0;
      state on
        entry:yjhx=1;
      (default) -> MANUAL.suoding.A
      MANUAL.suoding.on -> MANUAL.suoding.A : [suoding==0]
      MANUAL.suoding.A -> MANUAL.suoding.on : [suoding==1]
    state jiesuo [parallel]
      settings: executionOrder=6
      state A
        entry:skhx=0;
      state on
        entry:skhx=1;
      (default) -> MANUAL.jiesuo.A
      MANUAL.jiesuo.on -> MANUAL.jiesuo.A : [jiesuo==0]
      MANUAL.jiesuo.A -> MANUAL.jiesuo.on : [jiesuo==1]
  state off1
  state on1
    entry:
    skhx=0;
    kghx=0;
    yjhx=0;
    gghx=0;
  state end
    en:
    skhx=0;
    kghx=0;
    yjhx=0;
    gghx=0
  (default) -> off1
  off1 -> on1 : [tiaoshi==1]
  on1 -> MANUAL : after(500,tick)
  MANUAL -> end : [jiting==1]
  data: skhx output double; kghx output double; tiaoshi input double; songkai input; kaigai input; suoding input; jiesuo input; guangai input; yajin input; jiting input; yjhx output double; gghx output double
